simulink model "omc"  (Simulink 6.2)
settings: Solver=ode45  StartTime=0.0  StopTime=10.0  RelTol=1e-3
libraries: dsparch4 x38, cdsEpicsOut x29, Matrix8x x6, cdsOsc x5, dac x1, cdsPhase x1
settings Model: LastModifiedBy=rolf
settings DebuggingCC: SolverPrmCheckMsg=warning

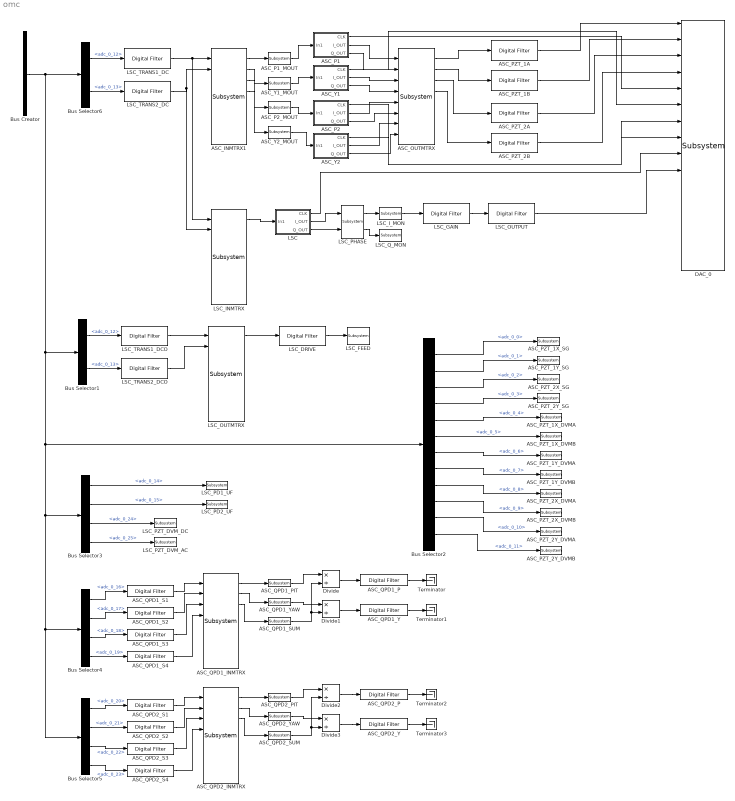
== system omc ==
  ASC_INMTRX1 : Matrix8x/Subsystem
  ASC_OUTMTRX : Matrix8x/Subsystem
  ASC_P1 : Subsystem
  ASC_P1_MOUT : cdsEpicsOut/Subsystem
  ASC_P2 : Subsystem
  ASC_P2_MOUT : cdsEpicsOut/Subsystem
  ASC_PZT_1A : dsparch4/Digital Filter  DialogController=dspDDGCreate  DialogControllerArgs=DataTag6  TypePopup=IIR (poles & zeros)  IIRFiltStruct=Direct form II transposed  AllPoleFiltStruct=Direct form  FIRFiltStruct=Direct form  CoeffSource=Specify via dialog  NumCoeffs=[1 2]  DenCoeffs=[1 0.1]  BiQuadCoeffs=[1 0.3 0.4 1 0.1 0.2]  LatticeCoeffs=[0.2 0.4]  denIgnore=on  FiltPerSampPopup=One filter per frame  IC=0  ICnum=0  ICden=0  roundingMode=Floor  overflowMode=off  ScaleValues=1  scaleValueFracLength=14  stageInFracLength=15  stageOutFracLength=15
  ASC_PZT_1B : dsparch4/Digital Filter  DialogController=dspDDGCreate  DialogControllerArgs=DataTag7  TypePopup=IIR (poles & zeros)  IIRFiltStruct=Direct form II transposed  AllPoleFiltStruct=Direct form  FIRFiltStruct=Direct form  CoeffSource=Specify via dialog  NumCoeffs=[1 2]  DenCoeffs=[1 0.1]  BiQuadCoeffs=[1 0.3 0.4 1 0.1 0.2]  LatticeCoeffs=[0.2 0.4]  denIgnore=on  FiltPerSampPopup=One filter per frame  IC=0  ICnum=0  ICden=0  roundingMode=Floor  overflowMode=off  ScaleValues=1  scaleValueFracLength=14  stageInFracLength=15  stageOutFracLength=15
  ASC_PZT_1X_DVMA : cdsEpicsOut/Subsystem
  ASC_PZT_1X_DVMB : cdsEpicsOut/Subsystem
  ASC_PZT_1X_SG : cdsEpicsOut/Subsystem
  ASC_PZT_1Y_DVMA : cdsEpicsOut/Subsystem
  ASC_PZT_1Y_DVMB : cdsEpicsOut/Subsystem
  ASC_PZT_1Y_SG : cdsEpicsOut/Subsystem
  ASC_PZT_2A : dsparch4/Digital Filter  DialogController=dspDDGCreate  DialogControllerArgs=DataTag8  TypePopup=IIR (poles & zeros)  IIRFiltStruct=Direct form II transposed  AllPoleFiltStruct=Direct form  FIRFiltStruct=Direct form  CoeffSource=Specify via dialog  NumCoeffs=[1 2]  DenCoeffs=[1 0.1]  BiQuadCoeffs=[1 0.3 0.4 1 0.1 0.2]  LatticeCoeffs=[0.2 0.4]  denIgnore=on  FiltPerSampPopup=One filter per frame  IC=0  ICnum=0  ICden=0  roundingMode=Floor  overflowMode=off  ScaleValues=1  scaleValueFracLength=14  stageInFracLength=15  stageOutFracLength=15
  ASC_PZT_2B : dsparch4/Digital Filter  DialogController=dspDDGCreate  DialogControllerArgs=DataTag9  TypePopup=IIR (poles & zeros)  IIRFiltStruct=Direct form II transposed  AllPoleFiltStruct=Direct form  FIRFiltStruct=Direct form  CoeffSource=Specify via dialog  NumCoeffs=[1 2]  DenCoeffs=[1 0.1]  BiQuadCoeffs=[1 0.3 0.4 1 0.1 0.2]  LatticeCoeffs=[0.2 0.4]  denIgnore=on  FiltPerSampPopup=One filter per frame  IC=0  ICnum=0  ICden=0  roundingMode=Floor  overflowMode=off  ScaleValues=1  scaleValueFracLength=14  stageInFracLength=15  stageOutFracLength=15
  ASC_PZT_2X_DVMA : cdsEpicsOut/Subsystem
  ASC_PZT_2X_DVMB : cdsEpicsOut/Subsystem
  ASC_PZT_2X_SG : cdsEpicsOut/Subsystem
  ASC_PZT_2Y_DVMA : cdsEpicsOut/Subsystem
  ASC_PZT_2Y_DVMB : cdsEpicsOut/Subsystem
  ASC_PZT_2Y_SG : cdsEpicsOut/Subsystem
  ASC_QPD1_INMTRX : Matrix8x/Subsystem
  ASC_QPD1_P : dsparch4/Digital Filter  DialogController=dspDDGCreate  DialogControllerArgs=DataTag10  TypePopup=IIR (poles & zeros)  IIRFiltStruct=Direct form II transposed  AllPoleFiltStruct=Direct form  FIRFiltStruct=Direct form  CoeffSource=Specify via dialog  NumCoeffs=[1 2]  DenCoeffs=[1 0.1]  BiQuadCoeffs=[1 0.3 0.4 1 0.1 0.2]  LatticeCoeffs=[0.2 0.4]  denIgnore=on  FiltPerSampPopup=One filter per frame  IC=0  ICnum=0  ICden=0  roundingMode=Floor  overflowMode=off  ScaleValues=1  scaleValueFracLength=14  stageInFracLength=15  stageOutFracLength=15
  ASC_QPD1_PIT : cdsEpicsOut/Subsystem
  ASC_QPD1_S1 : dsparch4/Digital Filter  DialogController=dspDDGCreate  DialogControllerArgs=DataTag11  TypePopup=IIR (poles & zeros)  IIRFiltStruct=Direct form II transposed  AllPoleFiltStruct=Direct form  FIRFiltStruct=Direct form  CoeffSource=Specify via dialog  NumCoeffs=[1 2]  DenCoeffs=[1 0.1]  BiQuadCoeffs=[1 0.3 0.4 1 0.1 0.2]  LatticeCoeffs=[0.2 0.4]  denIgnore=on  FiltPerSampPopup=One filter per frame  IC=0  ICnum=0  ICden=0  roundingMode=Floor  overflowMode=off  ScaleValues=1  scaleValueFracLength=14  stageInFracLength=15  stageOutFracLength=15
  ASC_QPD1_S2 : dsparch4/Digital Filter  DialogController=dspDDGCreate  DialogControllerArgs=DataTag12  TypePopup=IIR (poles & zeros)  IIRFiltStruct=Direct form II transposed  AllPoleFiltStruct=Direct form  FIRFiltStruct=Direct form  CoeffSource=Specify via dialog  NumCoeffs=[1 2]  DenCoeffs=[1 0.1]  BiQuadCoeffs=[1 0.3 0.4 1 0.1 0.2]  LatticeCoeffs=[0.2 0.4]  denIgnore=on  FiltPerSampPopup=One filter per frame  IC=0  ICnum=0  ICden=0  roundingMode=Floor  overflowMode=off  ScaleValues=1  scaleValueFracLength=14  stageInFracLength=15  stageOutFracLength=15
  ASC_QPD1_S3 : dsparch4/Digital Filter  DialogController=dspDDGCreate  DialogControllerArgs=DataTag13  TypePopup=IIR (poles & zeros)  IIRFiltStruct=Direct form II transposed  AllPoleFiltStruct=Direct form  FIRFiltStruct=Direct form  CoeffSource=Specify via dialog  NumCoeffs=[1 2]  DenCoeffs=[1 0.1]  BiQuadCoeffs=[1 0.3 0.4 1 0.1 0.2]  LatticeCoeffs=[0.2 0.4]  denIgnore=on  FiltPerSampPopup=One filter per frame  IC=0  ICnum=0  ICden=0  roundingMode=Floor  overflowMode=off  ScaleValues=1  scaleValueFracLength=14  stageInFracLength=15  stageOutFracLength=15
  ASC_QPD1_S4 : dsparch4/Digital Filter  DialogController=dspDDGCreate  DialogControllerArgs=DataTag14  TypePopup=IIR (poles & zeros)  IIRFiltStruct=Direct form II transposed  AllPoleFiltStruct=Direct form  FIRFiltStruct=Direct form  CoeffSource=Specify via dialog  NumCoeffs=[1 2]  DenCoeffs=[1 0.1]  BiQuadCoeffs=[1 0.3 0.4 1 0.1 0.2]  LatticeCoeffs=[0.2 0.4]  denIgnore=on  FiltPerSampPopup=One filter per frame  IC=0  ICnum=0  ICden=0  roundingMode=Floor  overflowMode=off  ScaleValues=1  scaleValueFracLength=14  stageInFracLength=15  stageOutFracLength=15
  ASC_QPD1_SUM : cdsEpicsOut/Subsystem
  ASC_QPD1_Y : dsparch4/Digital Filter  DialogController=dspDDGCreate  DialogControllerArgs=DataTag15  TypePopup=IIR (poles & zeros)  IIRFiltStruct=Direct form II transposed  AllPoleFiltStruct=Direct form  FIRFiltStruct=Direct form  CoeffSource=Specify via dialog  NumCoeffs=[1 2]  DenCoeffs=[1 0.1]  BiQuadCoeffs=[1 0.3 0.4 1 0.1 0.2]  LatticeCoeffs=[0.2 0.4]  denIgnore=on  FiltPerSampPopup=One filter per frame  IC=0  ICnum=0  ICden=0  roundingMode=Floor  overflowMode=off  ScaleValues=1  scaleValueFracLength=14  stageInFracLength=15  stageOutFracLength=15
  ASC_QPD1_YAW : cdsEpicsOut/Subsystem
  ASC_QPD2_INMTRX : Matrix8x/Subsystem
  ASC_QPD2_P : dsparch4/Digital Filter  DialogController=dspDDGCreate  DialogControllerArgs=DataTag16  TypePopup=IIR (poles & zeros)  IIRFiltStruct=Direct form II transposed  AllPoleFiltStruct=Direct form  FIRFiltStruct=Direct form  CoeffSource=Specify via dialog  NumCoeffs=[1 2]  DenCoeffs=[1 0.1]  BiQuadCoeffs=[1 0.3 0.4 1 0.1 0.2]  LatticeCoeffs=[0.2 0.4]  denIgnore=on  FiltPerSampPopup=One filter per frame  IC=0  ICnum=0  ICden=0  roundingMode=Floor  overflowMode=off  ScaleValues=1  scaleValueFracLength=14  stageInFracLength=15  stageOutFracLength=15
  ASC_QPD2_PIT : cdsEpicsOut/Subsystem
  ASC_QPD2_S1 : dsparch4/Digital Filter  DialogController=dspDDGCreate  DialogControllerArgs=DataTag17  TypePopup=IIR (poles & zeros)  IIRFiltStruct=Direct form II transposed  AllPoleFiltStruct=Direct form  FIRFiltStruct=Direct form  CoeffSource=Specify via dialog  NumCoeffs=[1 2]  DenCoeffs=[1 0.1]  BiQuadCoeffs=[1 0.3 0.4 1 0.1 0.2]  LatticeCoeffs=[0.2 0.4]  denIgnore=on  FiltPerSampPopup=One filter per frame  IC=0  ICnum=0  ICden=0  roundingMode=Floor  overflowMode=off  ScaleValues=1  scaleValueFracLength=14  stageInFracLength=15  stageOutFracLength=15
  ASC_QPD2_S2 : dsparch4/Digital Filter  DialogController=dspDDGCreate  DialogControllerArgs=DataTag18  TypePopup=IIR (poles & zeros)  IIRFiltStruct=Direct form II transposed  AllPoleFiltStruct=Direct form  FIRFiltStruct=Direct form  CoeffSource=Specify via dialog  NumCoeffs=[1 2]  DenCoeffs=[1 0.1]  BiQuadCoeffs=[1 0.3 0.4 1 0.1 0.2]  LatticeCoeffs=[0.2 0.4]  denIgnore=on  FiltPerSampPopup=One filter per frame  IC=0  ICnum=0  ICden=0  roundingMode=Floor  overflowMode=off  ScaleValues=1  scaleValueFracLength=14  stageInFracLength=15  stageOutFracLength=15
  ASC_QPD2_S3 : dsparch4/Digital Filter  DialogController=dspDDGCreate  DialogControllerArgs=DataTag19  TypePopup=IIR (poles & zeros)  IIRFiltStruct=Direct form II transposed  AllPoleFiltStruct=Direct form  FIRFiltStruct=Direct form  CoeffSource=Specify via dialog  NumCoeffs=[1 2]  DenCoeffs=[1 0.1]  BiQuadCoeffs=[1 0.3 0.4 1 0.1 0.2]  LatticeCoeffs=[0.2 0.4]  denIgnore=on  FiltPerSampPopup=One filter per frame  IC=0  ICnum=0  ICden=0  roundingMode=Floor  overflowMode=off  ScaleValues=1  scaleValueFracLength=14  stageInFracLength=15  stageOutFracLength=15
  ASC_QPD2_S4 : dsparch4/Digital Filter  DialogController=dspDDGCreate  DialogControllerArgs=DataTag20  TypePopup=IIR (poles & zeros)  IIRFiltStruct=Direct form II transposed  AllPoleFiltStruct=Direct form  FIRFiltStruct=Direct form  CoeffSource=Specify via dialog  NumCoeffs=[1 2]  DenCoeffs=[1 0.1]  BiQuadCoeffs=[1 0.3 0.4 1 0.1 0.2]  LatticeCoeffs=[0.2 0.4]  denIgnore=on  FiltPerSampPopup=One filter per frame  IC=0  ICnum=0  ICden=0  roundingMode=Floor  overflowMode=off  ScaleValues=1  scaleValueFracLength=14  stageInFracLength=15  stageOutFracLength=15
  ASC_QPD2_SUM : cdsEpicsOut/Subsystem
  ASC_QPD2_Y : dsparch4/Digital Filter  DialogController=dspDDGCreate  DialogControllerArgs=DataTag21  TypePopup=IIR (poles & zeros)  IIRFiltStruct=Direct form II transposed  AllPoleFiltStruct=Direct form  FIRFiltStruct=Direct form  CoeffSource=Specify via dialog  NumCoeffs=[1 2]  DenCoeffs=[1 0.1]  BiQuadCoeffs=[1 0.3 0.4 1 0.1 0.2]  LatticeCoeffs=[0.2 0.4]  denIgnore=on  FiltPerSampPopup=One filter per frame  IC=0  ICnum=0  ICden=0  roundingMode=Floor  overflowMode=off  ScaleValues=1  scaleValueFracLength=14  stageInFracLength=15  stageOutFracLength=15
  ASC_QPD2_YAW : cdsEpicsOut/Subsystem
  ASC_Y1 : Subsystem
  ASC_Y1_MOUT : cdsEpicsOut/Subsystem
  ASC_Y2 : Subsystem
  ASC_Y2_MOUT : cdsEpicsOut/Subsystem
  Bus Creator : BusCreator  Inputs='adc_0_0','adc_0_1','adc_0_2','adc_0_3','adc_0_4','adc_0_5','adc_0_6','adc_0_7','adc_0_8','adc_0_9','adc_0_10','adc_0_11','adc_0_12','adc_0_13','adc_0_14','adc_0_15','adc_0_16','adc_0_17','adc_0_18','adc_0_19','adc_0_20','adc_0_21','adc_0_22','adc_0_23','adc_0_24','adc_0_25','adc_0_26','adc_0_27','adc_0_28','adc_0_29','adc_0_30','adc_0_31'
  Bus Selector1 : BusSelector  OutputSignals=adc_0_12,adc_0_13
  Bus Selector2 : BusSelector  OutputSignals=adc_0_0,adc_0_1,adc_0_2,adc_0_3,adc_0_4,adc_0_5,adc_0_6,adc_0_7,adc_0_8,adc_0_9,adc_0_10,adc_0_11
  Bus Selector3 : BusSelector  OutputSignals=adc_0_14,adc_0_15,adc_0_24,adc_0_25
  Bus Selector4 : BusSelector  OutputSignals=adc_0_16,adc_0_17,adc_0_18,adc_0_19
  Bus Selector5 : BusSelector  OutputSignals=adc_0_20,adc_0_21,adc_0_22,adc_0_23
  Bus Selector6 : BusSelector  OutputSignals=adc_0_12,adc_0_13
  DAC_0 : dac/Subsystem
  Divide{,1..3} (4 alike) : Product  Inputs=*/  OutScaling=2^-10
  LSC : Subsystem
  LSC_DRIVE : dsparch4/Digital Filter  DialogController=dspDDGCreate  DialogControllerArgs=DataTag31  TypePopup=IIR (poles & zeros)  IIRFiltStruct=Direct form II transposed  AllPoleFiltStruct=Direct form  FIRFiltStruct=Direct form  CoeffSource=Specify via dialog  NumCoeffs=[1 2]  DenCoeffs=[1 0.1]  BiQuadCoeffs=[1 0.3 0.4 1 0.1 0.2]  LatticeCoeffs=[0.2 0.4]  denIgnore=on  FiltPerSampPopup=One filter per frame  IC=0  ICnum=0  ICden=0  roundingMode=Floor  overflowMode=off  ScaleValues=1  scaleValueFracLength=14  stageInFracLength=15  stageOutFracLength=15
  LSC_FEED : cdsEpicsOut/Subsystem
  LSC_GAIN : dsparch4/Digital Filter  DialogController=dspDDGCreate  DialogControllerArgs=DataTag32  TypePopup=IIR (poles & zeros)  IIRFiltStruct=Direct form II transposed  AllPoleFiltStruct=Direct form  FIRFiltStruct=Direct form  CoeffSource=Specify via dialog  NumCoeffs=[1 2]  DenCoeffs=[1 0.1]  BiQuadCoeffs=[1 0.3 0.4 1 0.1 0.2]  LatticeCoeffs=[0.2 0.4]  denIgnore=on  FiltPerSampPopup=One filter per frame  IC=0  ICnum=0  ICden=0  roundingMode=Floor  overflowMode=off  ScaleValues=1  scaleValueFracLength=14  stageInFracLength=15  stageOutFracLength=15
  LSC_INMTRX : Matrix8x/Subsystem
  LSC_I_MON : cdsEpicsOut/Subsystem
  LSC_OUTMTRX : Matrix8x/Subsystem
  LSC_OUTPUT : dsparch4/Digital Filter  DialogController=dspDDGCreate  DialogControllerArgs=DataTag33  TypePopup=IIR (poles & zeros)  IIRFiltStruct=Direct form II transposed  AllPoleFiltStruct=Direct form  FIRFiltStruct=Direct form  CoeffSource=Specify via dialog  NumCoeffs=[1 2]  DenCoeffs=[1 0.1]  BiQuadCoeffs=[1 0.3 0.4 1 0.1 0.2]  LatticeCoeffs=[0.2 0.4]  denIgnore=on  FiltPerSampPopup=One filter per frame  IC=0  ICnum=0  ICden=0  roundingMode=Floor  overflowMode=off  ScaleValues=1  scaleValueFracLength=14  stageInFracLength=15  stageOutFracLength=15
  LSC_PD1_UF : cdsEpicsOut/Subsystem
  LSC_PD2_UF : cdsEpicsOut/Subsystem
  LSC_PHASE : cdsPhase/Subsystem
  LSC_PZT_DVM_AC : cdsEpicsOut/Subsystem
  LSC_PZT_DVM_DC : cdsEpicsOut/Subsystem
  LSC_Q_MON : cdsEpicsOut/Subsystem
  LSC_TRANS1_DC : dsparch4/Digital Filter  DialogController=dspDDGCreate  DialogControllerArgs=DataTag34  TypePopup=IIR (poles & zeros)  IIRFiltStruct=Direct form II transposed  AllPoleFiltStruct=Direct form  FIRFiltStruct=Direct form  CoeffSource=Specify via dialog  NumCoeffs=[1 2]  DenCoeffs=[1 0.1]  BiQuadCoeffs=[1 0.3 0.4 1 0.1 0.2]  LatticeCoeffs=[0.2 0.4]  denIgnore=on  FiltPerSampPopup=One filter per frame  IC=0  ICnum=0  ICden=0  roundingMode=Floor  overflowMode=off  ScaleValues=1  scaleValueFracLength=14  stageInFracLength=15  stageOutFracLength=15
  LSC_TRANS1_DCO : dsparch4/Digital Filter  DialogController=dspDDGCreate  DialogControllerArgs=DataTag35  TypePopup=IIR (poles & zeros)  IIRFiltStruct=Direct form II transposed  AllPoleFiltStruct=Direct form  FIRFiltStruct=Direct form  CoeffSource=Specify via dialog  NumCoeffs=[1 2]  DenCoeffs=[1 0.1]  BiQuadCoeffs=[1 0.3 0.4 1 0.1 0.2]  LatticeCoeffs=[0.2 0.4]  denIgnore=on  FiltPerSampPopup=One filter per frame  IC=0  ICnum=0  ICden=0  roundingMode=Floor  overflowMode=off  ScaleValues=1  scaleValueFracLength=14  stageInFracLength=15  stageOutFracLength=15
  LSC_TRANS2_DC : dsparch4/Digital Filter  DialogController=dspDDGCreate  DialogControllerArgs=DataTag36  TypePopup=IIR (poles & zeros)  IIRFiltStruct=Direct form II transposed  AllPoleFiltStruct=Direct form  FIRFiltStruct=Direct form  CoeffSource=Specify via dialog  NumCoeffs=[1 2]  DenCoeffs=[1 0.1]  BiQuadCoeffs=[1 0.3 0.4 1 0.1 0.2]  LatticeCoeffs=[0.2 0.4]  denIgnore=on  FiltPerSampPopup=One filter per frame  IC=0  ICnum=0  ICden=0  roundingMode=Floor  overflowMode=off  ScaleValues=1  scaleValueFracLength=14  stageInFracLength=15  stageOutFracLength=15
  LSC_TRANS2_DCO : dsparch4/Digital Filter  DialogController=dspDDGCreate  DialogControllerArgs=DataTag37  TypePopup=IIR (poles & zeros)  IIRFiltStruct=Direct form II transposed  AllPoleFiltStruct=Direct form  FIRFiltStruct=Direct form  CoeffSource=Specify via dialog  NumCoeffs=[1 2]  DenCoeffs=[1 0.1]  BiQuadCoeffs=[1 0.3 0.4 1 0.1 0.2]  LatticeCoeffs=[0.2 0.4]  denIgnore=on  FiltPerSampPopup=One filter per frame  IC=0  ICnum=0  ICden=0  roundingMode=Floor  overflowMode=off  ScaleValues=1  scaleValueFracLength=14  stageInFracLength=15  stageOutFracLength=15
  Terminator{,1..3} (4 alike) : Terminator
  wires:
  Bus Creator/1 -> Bus Selector6/1, Bus Selector1/1, Bus Selector2/1, Bus Selector3/1, Bus Selector4/1, Bus Selector5/1
  Bus Selector6/1 -> LSC_TRANS1_DC/1  "<adc_0_12>"
  Bus Selector6/2 -> LSC_TRANS2_DC/1  "<adc_0_13>"
  LSC_PHASE/1 -> LSC_I_MON/1
  LSC_PHASE/2 -> LSC_Q_MON/1
  LSC_I_MON/1 -> LSC_GAIN/1
  LSC_GAIN/1 -> LSC_OUTPUT/1
  LSC_TRANS1_DCO/1 -> LSC_OUTMTRX/1
  LSC_TRANS2_DCO/1 -> LSC_OUTMTRX/2
  ASC_OUTMTRX/1 -> ASC_PZT_1A/1
  ASC_OUTMTRX/2 -> ASC_PZT_1B/1
  ASC_OUTMTRX/3 -> ASC_PZT_2A/1
  ASC_OUTMTRX/4 -> ASC_PZT_2B/1
  LSC_TRANS1_DC/1 -> ASC_INMTRX1/1, LSC_INMTRX/1
  LSC_TRANS2_DC/1 -> ASC_INMTRX1/2, LSC_INMTRX/2
  ASC_PZT_1A/1 -> DAC_0/1
  ASC_PZT_1B/1 -> DAC_0/2
  ASC_PZT_2A/1 -> DAC_0/3
  ASC_PZT_2B/1 -> DAC_0/4
  ASC_P1/2(I_OUT) -> ASC_OUTMTRX/1
  ASC_P1/3(Q_OUT) -> ASC_OUTMTRX/2
  ASC_Y1/2(I_OUT) -> ASC_OUTMTRX/3
  ASC_Y1/3(Q_OUT) -> ASC_OUTMTRX/4
  ASC_P2/2(I_OUT) -> ASC_OUTMTRX/5
  ASC_P2/3(Q_OUT) -> ASC_OUTMTRX/6
  ASC_Y2/2(I_OUT) -> ASC_OUTMTRX/7
  ASC_Y2/3(Q_OUT) -> ASC_OUTMTRX/8
  ASC_P1/1(CLK) -> DAC_0/5
  ASC_Y1/1(CLK) -> DAC_0/6
  ASC_P2/1(CLK) -> DAC_0/7
  ASC_Y2/1(CLK) -> DAC_0/8
  LSC_INMTRX/1 -> LSC/1(In1)
  LSC/2(I_OUT) -> LSC_PHASE/1
  LSC/3(Q_OUT) -> LSC_PHASE/2
  ASC_INMTRX1/1 -> ASC_P1_MOUT/1
  ASC_INMTRX1/2 -> ASC_Y1_MOUT/1
  ASC_INMTRX1/3 -> ASC_P2_MOUT/1
  ASC_INMTRX1/4 -> ASC_Y2_MOUT/1
  ASC_P1_MOUT/1 -> ASC_P1/1(In1)
  ASC_Y1_MOUT/1 -> ASC_Y1/1(In1)
  ASC_P2_MOUT/1 -> ASC_P2/1(In1)
  ASC_Y2_MOUT/1 -> ASC_Y2/1(In1)
  LSC_OUTMTRX/1 -> LSC_DRIVE/1
  LSC_DRIVE/1 -> LSC_FEED/1
  Bus Selector1/1 -> LSC_TRANS1_DCO/1  "<adc_0_12>"
  Bus Selector1/2 -> LSC_TRANS2_DCO/1  "<adc_0_13>"
  Bus Selector2/1 -> ASC_PZT_1X_SG/1  "<adc_0_0>"
  Bus Selector2/2 -> ASC_PZT_1Y_SG/1  "<adc_0_1>"
  Bus Selector2/3 -> ASC_PZT_2X_SG/1  "<adc_0_2>"
  Bus Selector2/4 -> ASC_PZT_2Y_SG/1  "<adc_0_3>"
  Bus Selector2/5 -> ASC_PZT_1X_DVMA/1  "<adc_0_4>"
  Bus Selector2/6 -> ASC_PZT_1X_DVMB/1  "<adc_0_5>"
  Bus Selector2/7 -> ASC_PZT_1Y_DVMA/1  "<adc_0_6>"
  Bus Selector2/8 -> ASC_PZT_1Y_DVMB/1  "<adc_0_7>"
  Bus Selector2/9 -> ASC_PZT_2X_DVMA/1  "<adc_0_8>"
  Bus Selector2/10 -> ASC_PZT_2X_DVMB/1  "<adc_0_9>"
  Bus Selector2/11 -> ASC_PZT_2Y_DVMA/1  "<adc_0_10>"
  Bus Selector2/12 -> ASC_PZT_2Y_DVMB/1  "<adc_0_11>"
  Bus Selector3/1 -> LSC_PD1_UF/1  "<adc_0_14>"
  Bus Selector3/2 -> LSC_PD2_UF/1  "<adc_0_15>"
  Bus Selector3/3 -> LSC_PZT_DVM_DC/1  "<adc_0_24>"
  Bus Selector3/4 -> LSC_PZT_DVM_AC/1  "<adc_0_25>"
  Bus Selector4/1 -> ASC_QPD1_S1/1  "<adc_0_16>"
  Bus Selector4/2 -> ASC_QPD1_S2/1  "<adc_0_17>"
  Bus Selector4/3 -> ASC_QPD1_S3/1  "<adc_0_18>"
  Bus Selector4/4 -> ASC_QPD1_S4/1  "<adc_0_19>"
  ASC_QPD1_S1/1 -> ASC_QPD1_INMTRX/1
  ASC_QPD1_S2/1 -> ASC_QPD1_INMTRX/2
  ASC_QPD1_S3/1 -> ASC_QPD1_INMTRX/3
  ASC_QPD1_S4/1 -> ASC_QPD1_INMTRX/4
  ASC_QPD2_S1/1 -> ASC_QPD2_INMTRX/1
  ASC_QPD2_S2/1 -> ASC_QPD2_INMTRX/2
  ASC_QPD2_S3/1 -> ASC_QPD2_INMTRX/3
  ASC_QPD2_S4/1 -> ASC_QPD2_INMTRX/4
  Bus Selector5/1 -> ASC_QPD2_S1/1  "<adc_0_20>"
  Bus Selector5/2 -> ASC_QPD2_S2/1  "<adc_0_21>"
  Bus Selector5/3 -> ASC_QPD2_S3/1  "<adc_0_22>"
  Bus Selector5/4 -> ASC_QPD2_S4/1  "<adc_0_23>"
  LSC/1(CLK) -> DAC_0/9
  LSC_OUTPUT/1 -> DAC_0/10
  ASC_QPD1_INMTRX/1 -> ASC_QPD1_PIT/1
  ASC_QPD1_INMTRX/2 -> ASC_QPD1_YAW/1
  ASC_QPD1_INMTRX/3 -> ASC_QPD1_SUM/1
  ASC_QPD1_PIT/1 -> Divide/1
  ASC_QPD1_YAW/1 -> Divide1/1
  ASC_QPD1_SUM/1 -> Divide/2, Divide1/2
  Divide/1 -> ASC_QPD1_P/1
  Divide1/1 -> ASC_QPD1_Y/1
  ASC_QPD1_P/1 -> Terminator/1
  ASC_QPD1_Y/1 -> Terminator1/1
  ASC_QPD2_PIT/1 -> Divide2/1
  ASC_QPD2_YAW/1 -> Divide3/1
  ASC_QPD2_SUM/1 -> Divide2/2, Divide3/2
  Divide2/1 -> ASC_QPD2_P/1
  Divide3/1 -> ASC_QPD2_Y/1
  ASC_QPD2_P/1 -> Terminator2/1
  ASC_QPD2_Y/1 -> Terminator3/1
  ASC_QPD2_INMTRX/1 -> ASC_QPD2_PIT/1
  ASC_QPD2_INMTRX/2 -> ASC_QPD2_YAW/1
  ASC_QPD2_INMTRX/3 -> ASC_QPD2_SUM/1

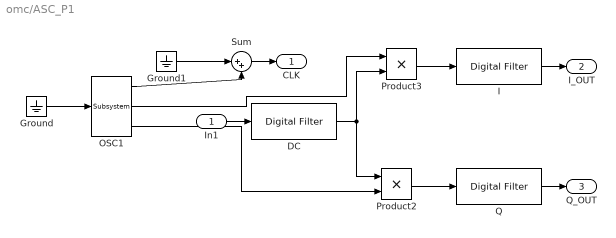
== system omc/ASC_P1 ==
  In1 : Inport  Port=1  LatchInput=off
  DC : dsparch4/Digital Filter  DialogController=dspDDGCreate  DialogControllerArgs=DataTag0  TypePopup=IIR (poles & zeros)  IIRFiltStruct=Direct form II transposed  AllPoleFiltStruct=Direct form  FIRFiltStruct=Direct form  CoeffSource=Specify via dialog  NumCoeffs=[1 2]  DenCoeffs=[1 0.1]  BiQuadCoeffs=[1 0.3 0.4 1 0.1 0.2]  LatticeCoeffs=[0.2 0.4]  denIgnore=on  FiltPerSampPopup=One filter per frame  IC=0  ICnum=0  ICden=0  roundingMode=Floor  overflowMode=off  ScaleValues=1  scaleValueFracLength=14  stageInFracLength=15  stageOutFracLength=15
  Ground : Ground
  Ground1 : Ground
  I : dsparch4/Digital Filter  DialogController=dspDDGCreate  DialogControllerArgs=DataTag1  TypePopup=IIR (poles & zeros)  IIRFiltStruct=Direct form II transposed  AllPoleFiltStruct=Direct form  FIRFiltStruct=Direct form  CoeffSource=Specify via dialog  NumCoeffs=[1 2]  DenCoeffs=[1 0.1]  BiQuadCoeffs=[1 0.3 0.4 1 0.1 0.2]  LatticeCoeffs=[0.2 0.4]  denIgnore=on  FiltPerSampPopup=One filter per frame  IC=0  ICnum=0  ICden=0  roundingMode=Floor  overflowMode=off  ScaleValues=1  scaleValueFracLength=14  stageInFracLength=15  stageOutFracLength=15
  OSC1 : cdsOsc/Subsystem
  Product2 : Product  RndMeth=Zero
  Product3 : Product  RndMeth=Zero
  Q : dsparch4/Digital Filter  DialogController=dspDDGCreate  DialogControllerArgs=DataTag2  TypePopup=IIR (poles & zeros)  IIRFiltStruct=Direct form II transposed  AllPoleFiltStruct=Direct form  FIRFiltStruct=Direct form  CoeffSource=Specify via dialog  NumCoeffs=[1 2]  DenCoeffs=[1 0.1]  BiQuadCoeffs=[1 0.3 0.4 1 0.1 0.2]  LatticeCoeffs=[0.2 0.4]  denIgnore=on  FiltPerSampPopup=One filter per frame  IC=0  ICnum=0  ICden=0  roundingMode=Floor  overflowMode=off  ScaleValues=1  scaleValueFracLength=14  stageInFracLength=15  stageOutFracLength=15
  Sum : Sum  Inputs=|++
  CLK : Outport
  I_OUT : Outport  Port=2
  Q_OUT : Outport  Port=3
  wires:
  DC/1 -> Product3/2, Product2/1
  Product3/1 -> I/1
  Product2/1 -> Q/1
  Ground/1 -> OSC1/1
  OSC1/1 -> Sum/2
  Ground1/1 -> Sum/1
  OSC1/2 -> Product3/1
  OSC1/3 -> Product2/2
  Sum/1 -> CLK/1
  I/1 -> I_OUT/1
  In1/1 -> DC/1
  Q/1 -> Q_OUT/1

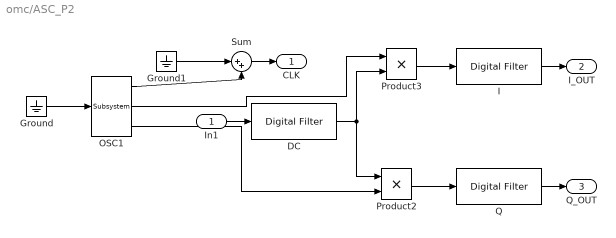
== system omc/ASC_P2 ==
  In1 : Inport  Port=1  LatchInput=off
  DC : dsparch4/Digital Filter  DialogController=dspDDGCreate  DialogControllerArgs=DataTag3  TypePopup=IIR (poles & zeros)  IIRFiltStruct=Direct form II transposed  AllPoleFiltStruct=Direct form  FIRFiltStruct=Direct form  CoeffSource=Specify via dialog  NumCoeffs=[1 2]  DenCoeffs=[1 0.1]  BiQuadCoeffs=[1 0.3 0.4 1 0.1 0.2]  LatticeCoeffs=[0.2 0.4]  denIgnore=on  FiltPerSampPopup=One filter per frame  IC=0  ICnum=0  ICden=0  roundingMode=Floor  overflowMode=off  ScaleValues=1  scaleValueFracLength=14  stageInFracLength=15  stageOutFracLength=15
  Ground : Ground
  Ground1 : Ground
  I : dsparch4/Digital Filter  DialogController=dspDDGCreate  DialogControllerArgs=DataTag4  TypePopup=IIR (poles & zeros)  IIRFiltStruct=Direct form II transposed  AllPoleFiltStruct=Direct form  FIRFiltStruct=Direct form  CoeffSource=Specify via dialog  NumCoeffs=[1 2]  DenCoeffs=[1 0.1]  BiQuadCoeffs=[1 0.3 0.4 1 0.1 0.2]  LatticeCoeffs=[0.2 0.4]  denIgnore=on  FiltPerSampPopup=One filter per frame  IC=0  ICnum=0  ICden=0  roundingMode=Floor  overflowMode=off  ScaleValues=1  scaleValueFracLength=14  stageInFracLength=15  stageOutFracLength=15
  OSC1 : cdsOsc/Subsystem
  Product2 : Product  RndMeth=Zero
  Product3 : Product  RndMeth=Zero
  Q : dsparch4/Digital Filter  DialogController=dspDDGCreate  DialogControllerArgs=DataTag5  TypePopup=IIR (poles & zeros)  IIRFiltStruct=Direct form II transposed  AllPoleFiltStruct=Direct form  FIRFiltStruct=Direct form  CoeffSource=Specify via dialog  NumCoeffs=[1 2]  DenCoeffs=[1 0.1]  BiQuadCoeffs=[1 0.3 0.4 1 0.1 0.2]  LatticeCoeffs=[0.2 0.4]  denIgnore=on  FiltPerSampPopup=One filter per frame  IC=0  ICnum=0  ICden=0  roundingMode=Floor  overflowMode=off  ScaleValues=1  scaleValueFracLength=14  stageInFracLength=15  stageOutFracLength=15
  Sum : Sum  Inputs=|++
  CLK : Outport
  I_OUT : Outport  Port=2
  Q_OUT : Outport  Port=3
  wires:
  DC/1 -> Product3/2, Product2/1
  Product3/1 -> I/1
  Product2/1 -> Q/1
  Ground/1 -> OSC1/1
  OSC1/1 -> Sum/2
  Ground1/1 -> Sum/1
  OSC1/2 -> Product3/1
  OSC1/3 -> Product2/2
  Sum/1 -> CLK/1
  I/1 -> I_OUT/1
  In1/1 -> DC/1
  Q/1 -> Q_OUT/1

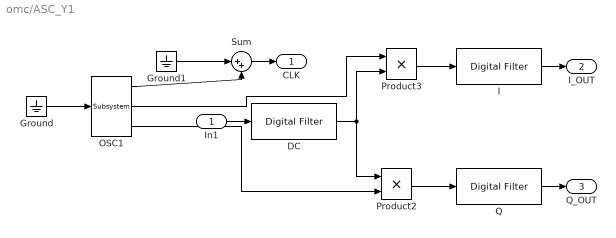
== system omc/ASC_Y1 ==
  In1 : Inport  Port=1  LatchInput=off
  DC : dsparch4/Digital Filter  DialogController=dspDDGCreate  DialogControllerArgs=DataTag22  TypePopup=IIR (poles & zeros)  IIRFiltStruct=Direct form II transposed  AllPoleFiltStruct=Direct form  FIRFiltStruct=Direct form  CoeffSource=Specify via dialog  NumCoeffs=[1 2]  DenCoeffs=[1 0.1]  BiQuadCoeffs=[1 0.3 0.4 1 0.1 0.2]  LatticeCoeffs=[0.2 0.4]  denIgnore=on  FiltPerSampPopup=One filter per frame  IC=0  ICnum=0  ICden=0  roundingMode=Floor  overflowMode=off  ScaleValues=1  scaleValueFracLength=14  stageInFracLength=15  stageOutFracLength=15
  Ground : Ground
  Ground1 : Ground
  I : dsparch4/Digital Filter  DialogController=dspDDGCreate  DialogControllerArgs=DataTag23  TypePopup=IIR (poles & zeros)  IIRFiltStruct=Direct form II transposed  AllPoleFiltStruct=Direct form  FIRFiltStruct=Direct form  CoeffSource=Specify via dialog  NumCoeffs=[1 2]  DenCoeffs=[1 0.1]  BiQuadCoeffs=[1 0.3 0.4 1 0.1 0.2]  LatticeCoeffs=[0.2 0.4]  denIgnore=on  FiltPerSampPopup=One filter per frame  IC=0  ICnum=0  ICden=0  roundingMode=Floor  overflowMode=off  ScaleValues=1  scaleValueFracLength=14  stageInFracLength=15  stageOutFracLength=15
  OSC1 : cdsOsc/Subsystem
  Product2 : Product  RndMeth=Zero
  Product3 : Product  RndMeth=Zero
  Q : dsparch4/Digital Filter  DialogController=dspDDGCreate  DialogControllerArgs=DataTag24  TypePopup=IIR (poles & zeros)  IIRFiltStruct=Direct form II transposed  AllPoleFiltStruct=Direct form  FIRFiltStruct=Direct form  CoeffSource=Specify via dialog  NumCoeffs=[1 2]  DenCoeffs=[1 0.1]  BiQuadCoeffs=[1 0.3 0.4 1 0.1 0.2]  LatticeCoeffs=[0.2 0.4]  denIgnore=on  FiltPerSampPopup=One filter per frame  IC=0  ICnum=0  ICden=0  roundingMode=Floor  overflowMode=off  ScaleValues=1  scaleValueFracLength=14  stageInFracLength=15  stageOutFracLength=15
  Sum : Sum  Inputs=|++
  CLK : Outport
  I_OUT : Outport  Port=2
  Q_OUT : Outport  Port=3
  wires:
  DC/1 -> Product3/2, Product2/1
  Product3/1 -> I/1
  Product2/1 -> Q/1
  Ground/1 -> OSC1/1
  OSC1/1 -> Sum/2
  Ground1/1 -> Sum/1
  OSC1/2 -> Product3/1
  OSC1/3 -> Product2/2
  Sum/1 -> CLK/1
  I/1 -> I_OUT/1
  In1/1 -> DC/1
  Q/1 -> Q_OUT/1

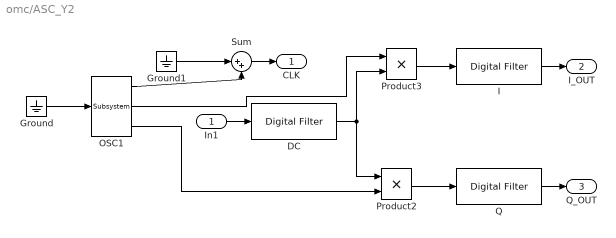
== system omc/ASC_Y2 ==
  In1 : Inport  Port=1  LatchInput=off
  DC : dsparch4/Digital Filter  DialogController=dspDDGCreate  DialogControllerArgs=DataTag25  TypePopup=IIR (poles & zeros)  IIRFiltStruct=Direct form II transposed  AllPoleFiltStruct=Direct form  FIRFiltStruct=Direct form  CoeffSource=Specify via dialog  NumCoeffs=[1 2]  DenCoeffs=[1 0.1]  BiQuadCoeffs=[1 0.3 0.4 1 0.1 0.2]  LatticeCoeffs=[0.2 0.4]  denIgnore=on  FiltPerSampPopup=One filter per frame  IC=0  ICnum=0  ICden=0  roundingMode=Floor  overflowMode=off  ScaleValues=1  scaleValueFracLength=14  stageInFracLength=15  stageOutFracLength=15
  Ground : Ground
  Ground1 : Ground
  I : dsparch4/Digital Filter  DialogController=dspDDGCreate  DialogControllerArgs=DataTag26  TypePopup=IIR (poles & zeros)  IIRFiltStruct=Direct form II transposed  AllPoleFiltStruct=Direct form  FIRFiltStruct=Direct form  CoeffSource=Specify via dialog  NumCoeffs=[1 2]  DenCoeffs=[1 0.1]  BiQuadCoeffs=[1 0.3 0.4 1 0.1 0.2]  LatticeCoeffs=[0.2 0.4]  denIgnore=on  FiltPerSampPopup=One filter per frame  IC=0  ICnum=0  ICden=0  roundingMode=Floor  overflowMode=off  ScaleValues=1  scaleValueFracLength=14  stageInFracLength=15  stageOutFracLength=15
  OSC1 : cdsOsc/Subsystem
  Product2 : Product  RndMeth=Zero
  Product3 : Product  RndMeth=Zero
  Q : dsparch4/Digital Filter  DialogController=dspDDGCreate  DialogControllerArgs=DataTag27  TypePopup=IIR (poles & zeros)  IIRFiltStruct=Direct form II transposed  AllPoleFiltStruct=Direct form  FIRFiltStruct=Direct form  CoeffSource=Specify via dialog  NumCoeffs=[1 2]  DenCoeffs=[1 0.1]  BiQuadCoeffs=[1 0.3 0.4 1 0.1 0.2]  LatticeCoeffs=[0.2 0.4]  denIgnore=on  FiltPerSampPopup=One filter per frame  IC=0  ICnum=0  ICden=0  roundingMode=Floor  overflowMode=off  ScaleValues=1  scaleValueFracLength=14  stageInFracLength=15  stageOutFracLength=15
  Sum : Sum  Inputs=|++
  CLK : Outport
  I_OUT : Outport  Port=2
  Q_OUT : Outport  Port=3
  wires:
  DC/1 -> Product3/2, Product2/1
  Product3/1 -> I/1
  Product2/1 -> Q/1
  Ground/1 -> OSC1/1
  OSC1/1 -> Sum/2
  Ground1/1 -> Sum/1
  OSC1/2 -> Product3/1
  OSC1/3 -> Product2/2
  Sum/1 -> CLK/1
  I/1 -> I_OUT/1
  In1/1 -> DC/1
  Q/1 -> Q_OUT/1

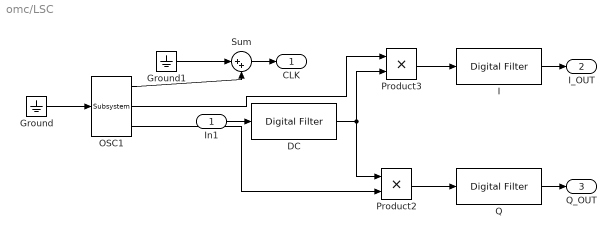
== system omc/LSC ==
  In1 : Inport  Port=1  LatchInput=off
  DC : dsparch4/Digital Filter  DialogController=dspDDGCreate  DialogControllerArgs=DataTag28  TypePopup=IIR (poles & zeros)  IIRFiltStruct=Direct form II transposed  AllPoleFiltStruct=Direct form  FIRFiltStruct=Direct form  CoeffSource=Specify via dialog  NumCoeffs=[1 2]  DenCoeffs=[1 0.1]  BiQuadCoeffs=[1 0.3 0.4 1 0.1 0.2]  LatticeCoeffs=[0.2 0.4]  denIgnore=on  FiltPerSampPopup=One filter per frame  IC=0  ICnum=0  ICden=0  roundingMode=Floor  overflowMode=off  ScaleValues=1  scaleValueFracLength=14  stageInFracLength=15  stageOutFracLength=15
  Ground : Ground
  Ground1 : Ground
  I : dsparch4/Digital Filter  DialogController=dspDDGCreate  DialogControllerArgs=DataTag29  TypePopup=IIR (poles & zeros)  IIRFiltStruct=Direct form II transposed  AllPoleFiltStruct=Direct form  FIRFiltStruct=Direct form  CoeffSource=Specify via dialog  NumCoeffs=[1 2]  DenCoeffs=[1 0.1]  BiQuadCoeffs=[1 0.3 0.4 1 0.1 0.2]  LatticeCoeffs=[0.2 0.4]  denIgnore=on  FiltPerSampPopup=One filter per frame  IC=0  ICnum=0  ICden=0  roundingMode=Floor  overflowMode=off  ScaleValues=1  scaleValueFracLength=14  stageInFracLength=15  stageOutFracLength=15
  OSC1 : cdsOsc/Subsystem
  Product2 : Product  RndMeth=Zero
  Product3 : Product  RndMeth=Zero
  Q : dsparch4/Digital Filter  DialogController=dspDDGCreate  DialogControllerArgs=DataTag30  TypePopup=IIR (poles & zeros)  IIRFiltStruct=Direct form II transposed  AllPoleFiltStruct=Direct form  FIRFiltStruct=Direct form  CoeffSource=Specify via dialog  NumCoeffs=[1 2]  DenCoeffs=[1 0.1]  BiQuadCoeffs=[1 0.3 0.4 1 0.1 0.2]  LatticeCoeffs=[0.2 0.4]  denIgnore=on  FiltPerSampPopup=One filter per frame  IC=0  ICnum=0  ICden=0  roundingMode=Floor  overflowMode=off  ScaleValues=1  scaleValueFracLength=14  stageInFracLength=15  stageOutFracLength=15
  Sum : Sum  Inputs=|++
  CLK : Outport
  I_OUT : Outport  Port=2
  Q_OUT : Outport  Port=3
  wires:
  DC/1 -> Product3/2, Product2/1
  Product3/1 -> I/1
  Product2/1 -> Q/1
  Ground/1 -> OSC1/1
  OSC1/1 -> Sum/2
  Ground1/1 -> Sum/1
  OSC1/2 -> Product3/1
  OSC1/3 -> Product2/2
  Sum/1 -> CLK/1
  I/1 -> I_OUT/1
  In1/1 -> DC/1
  Q/1 -> Q_OUT/1
